simulink model "beamforming_ofdm_phase_ura2"  (R2020b)
settings: Solver=VariableStepAuto  StartTime=0.0  StopTime=10^-6  RelTol=1e-3
undefined symbols (not defined in the file or in its folder): phased, physconst
libraries: commrandsrc3 x1, dspsigops x1, dspxfrm3 x1, dspindex x1, phasedbflib x1, eeGeneralControl x1
settings Model: Creator=Lakshmi Mounika  LastModifiedBy=Lakshmi Mounika

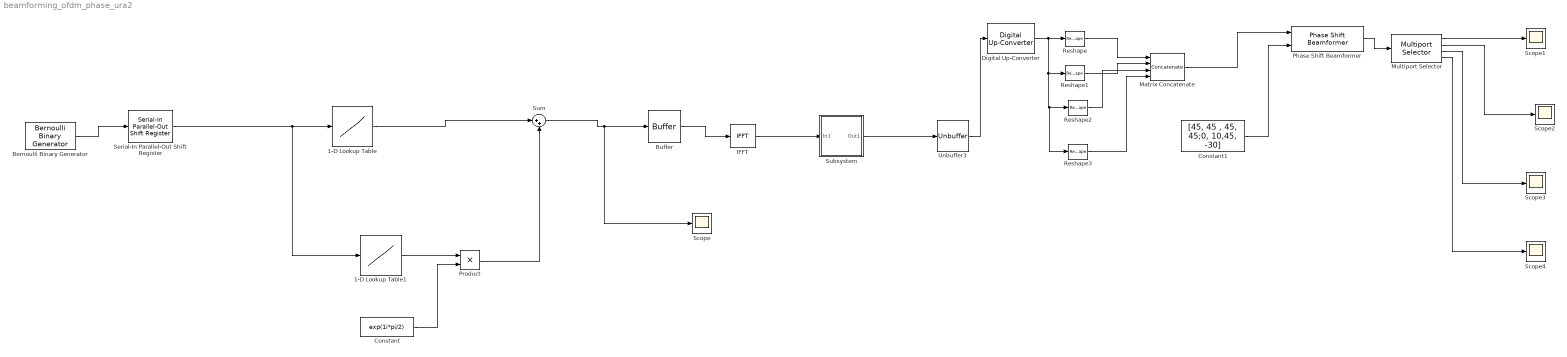
== system beamforming_ofdm_phase_ura2 ==
  1-D Lookup Table : Lookup_n-D  NumberOfTableDimensions=1  BreakpointsForDimension1=[0:3]  Table=[1, 1, -1, -1]  InternalRulePriority=Speed  RndMeth=Simplest  InputSameDT=on
  1-D Lookup Table1 : Lookup_n-D  NumberOfTableDimensions=1  BreakpointsForDimension1=[0:3]  Table=[1, -1, 1, -1]  InternalRulePriority=Speed  RndMeth=Simplest  InputSameDT=on
  Bernoulli Binary Generator : commrandsrc3/Bernoulli Binary Generator  ProbabilityOfZero=0.5  SeedSource=Parameter  Seed=61  SampleTime=0.05e-6  SamplesPerFrame=64  OutputDataType=boolean  SimulateUsing=Interpreted execution
  Buffer : Buffer  N=16  OutputFrames=off
  Constant : Constant  Value=exp(1i*pi/2)
  Constant1 : Constant  Value=[45, 45 , 45, 45;0, 10,45, -30]
  Digital Up-Converter : dspsigops/Digital Up-Converter  InterpolationFactor=100  MinimumOrderDesign=on  FirstFilterOrder=10  SecondFilterOrder=12  NumCICSections=3  Bandwidth=40e6  StopbandFrequencySource=Auto  StopbandFrequency=150000  PassbandRipple=0.1  StopbandAttenuation=60  Oscillator=Sine wave  CenterFrequency=800e6  NumAccumulatorBits=16  NumQuantizedAccumulatorBits=12  Dither=on  NumDitherBits=4  InheritSampleRate=on  SampleRate=800e6  SimulateUsing=Code generation  outputMin=[]  outputMax=[]
      settings: SourceProductBaseCode=DS
  IFFT : dspxfrm3/IFFT  FFTImplementation=Auto  CompMethod=Table lookup  TableOpt=NEW  TableOptActive=Speed  BitRevOrder=off  cs_in=off  Normalize=on  InheritFFTLength=off  FFTLength=64  WrapInput=on  mode=Complex  outSamplingMode=Sample based  roundingMode=Floor  overflowMode=off  firstCoeffDataTypeStr=Inherit: Same word length as input  firstCoeffLastDataTypeStr=Inherit: Same word length as input  outputMin=[]  outputMax=[]
  Matrix Concatenate : Concatenate  NumInputs=4  Mode=Multidimensional array  ConcatenateDimension=2
  Multiport Selector : dspindex/Multiport Selector  rowsOrCols=Columns  idxCellArray={1,2,3,4}  idxErrMode=Clip Index
  Phase Shift Beamformer : phasedbflib/Phase Shift Beamformer  PropagationSpeed=physconst( 'LightSpeed' )  OperatingFrequency=800e6  DirectionSource=Input port  Direction="45  (0, 45, 90, -45 )]"  NumPhaseShifterBits=0  WeightsNormalization=Distortionless  WeightsOutputPort=off  SimulateUsing=Interpreted execution  SensorArray=phased.URA('Size',[ 2, 2 ],'Element',phased.CustomAntennaElement('MatchArrayNormal',true,'FrequencyVector',[ 0, 800e6 ]),'ArrayNormal','y')
      settings: SourceProductBaseCode=AR
  Product : Product
  Reshape{,1..3} (4 alike) : Reshape  OutputDimensionality=Customize  OutputDimensions=[100]
  Scope{,1..4} (5 alike) : Scope
  Serial-In Parallel-Out Shift Register : eeGeneralControl/Serial-In Parallel-Out Shift Register  N=2  IC=0  Ts=-1
      settings: SourceProductBaseCode=PS
  Subsystem : Subsystem
      mask Display: disp('Add\nCyclic Prefix')
  Sum : Sum  Inputs=|++
  Unbuffer3 : Unbuffer
  wires:
  Multiport Selector/1 -> Scope1/1
  Product/1 -> Sum/2
  IFFT/1 -> Subsystem/1(In1)
  Subsystem/1(Out1) -> Unbuffer3/1
  Multiport Selector/3 -> Scope3/1
  Multiport Selector/4 -> Scope4/1
  Phase Shift Beamformer/1 -> Multiport Selector/1
  Multiport Selector/2 -> Scope2/1
  Serial-In Parallel-Out Shift Register/1 -> 1-D Lookup Table1/1, 1-D Lookup Table/1
  Buffer/1 -> IFFT/1
  1-D Lookup Table1/1 -> Product/1
  Sum/1 -> Scope/1, Buffer/1
  Reshape3/1 -> Matrix Concatenate/4
  Reshape/1 -> Matrix Concatenate/1
  Matrix Concatenate/1 -> Phase Shift Beamformer/1
  Unbuffer3/1 -> Digital Up-Converter/1
  Bernoulli Binary Generator/1 -> Serial-In Parallel-Out Shift Register/1
  Reshape1/1 -> Matrix Concatenate/2
  Reshape2/1 -> Matrix Concatenate/3
  Constant/1 -> Product/2
  Digital Up-Converter/1 -> Reshape3/1, Reshape2/1, Reshape1/1, Reshape/1
  1-D Lookup Table/1 -> Sum/1
  Constant1/1 -> Phase Shift Beamformer/2

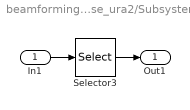
== system beamforming_ofdm_phase_ura2/Subsystem ==
  In1 : Inport
  Selector3 : Selector  NumberOfDimensions=2  InputPortWidth=64  IndexOptions=Index vector (dialog),Select all  Indices=[48:64,1:64],-1  OutputSizes=1
  Out1 : Outport
  wires:
  Selector3/1 -> Out1/1
  In1/1 -> Selector3/1
